simulink model "DTU_Topology_Long_Line"  (R2023b)
settings: Solver=ode4  StartTime=0.0  StopTime=stoptime  FixedStep=Ts  RelTol=1e-3
PreLoadFcn:
  | Ts=1e-4;run('Grid_Parameters_3ph.m');load('Data_3ph_Pars.mat');load('First_Busbar_Pars.mat');run('line_parameters.m')
PostLoadFcn:
  | Ts=1e-4;run('Grid_Parameters_3ph.m');load('Data_3ph_Pars.mat');load('First_Busbar_Pars.mat');run('line_parameters.m')
InitFcn:
  | Ts=1e-4;run('Grid_Parameters_3ph.m');load('Data_3ph_Pars.mat');load('First_Busbar_Pars.mat');run('line_parameters.m')
StartFcn:
  | Ts=1e-4;run('Grid_Parameters_3ph.m');load('Data_3ph_Pars.mat');load('First_Busbar_Pars.mat');run('line_parameters.m')
values from neighbouring files (symbols this model uses):
  datastart = 100    [Grid_Parameters_3ph.m]
  datastop = 700    [Grid_Parameters_3ph.m]
  fnom = 50    [Grid_Parameters_3ph.m]    (also in line_parameters.m)
  line_param = struct()    [line_parameters.m]
  t_factor = 1/acceleration    (= 1)    [Grid_Parameters_3ph.m]
  timestep_meas_data = 1    [Grid_Parameters_3ph.m]
  Vnom = 400    [Grid_Parameters_3ph.m]
undefined symbols (not defined in the file or in its folder): another_event_name, Data_3ph_Pars, First_Busbar_Pars, j, my_event_name, Newton, Raphson
libraries: spsSeriesRLCBranchLib x90, spsGroundLib x47, spsThreePhaseVIMeasurementLib x11, spsMutualInductanceLib x7, spsThreePhaseSineGeneratorLib x6, spsControlledVoltageSourceLib x3, spsControlledCurrentSourceLib x3, spsMeanLib x3, rtlab x2, spsThreePhaseSourceLib x1, spsThreePhaseSeriesRLCBranchLib x1, sps_lib x1
(part 1 of 2)
Description:
  | Model of a simple control system for use iin training.
settings Model: VariantFading=off  Creator=Alex  LastModifiedBy=obus
settings SolverCC: AlgebraicLoopSolver=TrustRegion  AutoInsertRateTranBlk=on
settings DataIOCC: LimitDataPoints=on  SaveFormat=Array  SignalLoggingSaveFormat=ModelDataLogs  SaveOutput=off  SaveTime=off  ReturnWorkspaceOutputs=off  SignalLoggingName=sigsOut
settings OptimizationCC: BlockReduction=off  BooleanDataType=off  OptimizeBlockIOStorage=off  BufferReuse=off  GlobalBufferReuse=off  ExpressionFolding=off  LocalBlockOutputs=off  InitFltsAndDblsToZero=on  LifeSpan=inf  OptimizeDataStoreBuffers=off  BusAssignmentInplaceUpdate=off
settings DebuggingCC: SaveWithParameterizedLinksMsg=none  UnderspecifiedInitializationDetection=Classic  MergeDetectMultiDrivingBlocksExec=none  SignalResolutionControl=TryResolveAllWithWarning  MultiTaskDSMMsg=warning  MultiTaskCondExecSysMsg=none  FcnCallInpInsideContextMsg=warning  UnconnectedInputMsg=warning  UnconnectedOutputMsg=warning  UnconnectedLineMsg=warning  SFUnexpectedBacktrackingDiag=warning  SFNoUnconditionalDefaultTransitionDiag=warning  SFExecutionAtInitializationDiag=none  ArithmeticOperatorsInVariantConditions=warning
settings HardwareCC: ProdBitPerPointer=32  ProdBitPerSizeT=32  ProdBitPerPtrDiffT=32  ProdLargestAtomicFloat=None  ProdIntDivRoundTo=Undefined  ProdEndianess=Unspecified  ProdWordSize=32  ProdHWDeviceType=32-bit Generic  TargetUnknown=on
settings ModelReferenceCC: EnableRefExpFcnMdlSchedulingChecks=on  PropagateSignalLabelsOutOfModel=off
settings SFSimCC: SimUseLocalCustomCode=off  CustomCodeUndefinedFunction=UseInterfaceOnly
settings RTWCC: RTWUseLocalCustomCode=off  DLArmComputeVersion=19.05
settings CodeAppCC: StateflowObjectComments=on
settings GRTTargetCC: TargetFcnLib=ansi_tfl_tmw.mat  TargetLangStandard=C89/C90 (ANSI)  CombineOutputUpdateFcns=off  GRTInterface=on
settings ConfigComp: CovMetricSettings=dw  CovSaveCumulativeToWorkspaceVar=on  CovSaveSingleToWorkspaceVar=on  CovExternalEMLEnable=off

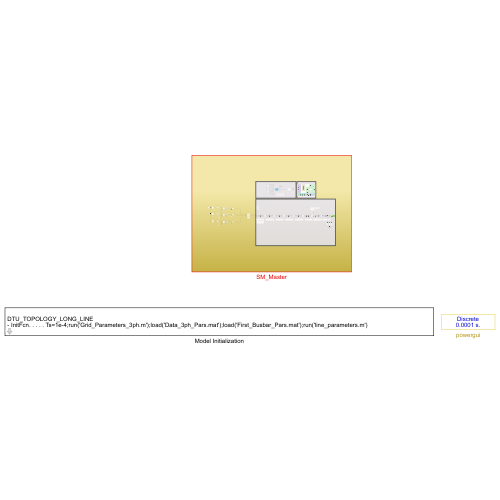
[thumbnail: Simulink's stored preview of the top-level diagram]
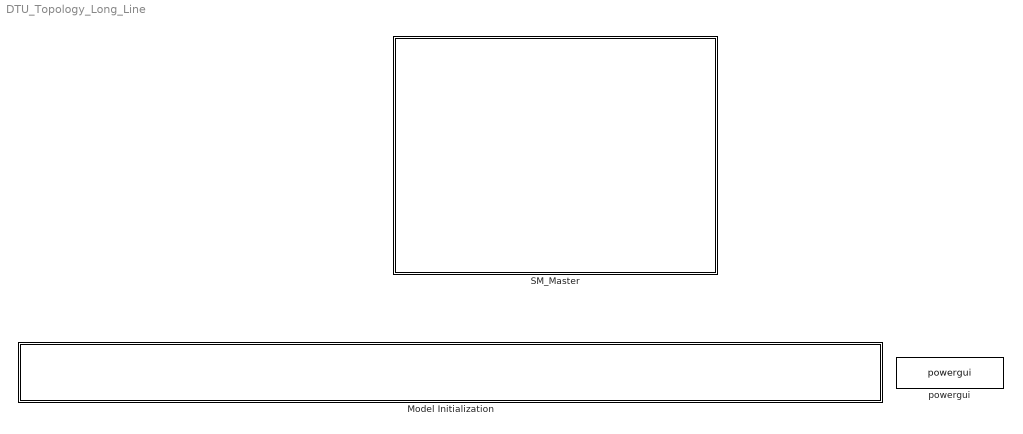
== system DTU_Topology_Long_Line ==
  Model Initialization : Subsystem  mask(Model Functions){InitFcnX=Ts=1e-4;run('Grid_Parameters_3ph.m');load('Data_3ph_Pars.mat');load('First_Busbar_Pars.mat');run('line_parameters.m'), prel=on, posl=on, inif=on, strf=on}
      mask prompts: InitFcnX "Initialisation"; prel "Preload Function"; posl "PostLoad Function"; inif "InitFcn"; strf "StartFcn"
      mask init:
      | currentBlock = gcb;
      | root = bdroot(currentBlock);
      | 
      | if ~strcmp(get_param(root,'BlockDiagramType'),'library')
      |     if prel==1
      |         set_param(root, 'PreLoadFcn', InitFcnX);
      |     else
      |         set_param(root, 'PreLoadFcn', '');
      |     end
      |     if inif==1
      |         set_param(root, 'InitFcn', InitFcnX);
      |     else
      |         set_param(root, 'InitFcn', '');
      |     end
      |     if strf==1
      |         set_param(root, 'StartFcn', InitFcnX);
      |     else
      |         set_param(root, 'StartFcn', '');
      |     end
      |     if posl==1
      |         set_param(root, 'PostLoadFcn', InitFcnX);
      |     else
      |         set_param(root, 'PostLoadFcn', '');
      |     end
      | end
      | 
      | pos = get_param(currentBlock, 'Position');
      | width = pos(3) - pos(1); height = pos(4) - pos(2);
      | txt = [ upper(root) '\n' '- InitFcn. . . . . '  get_param(root, 'InitFcn') ];
      settings: CopyFcn=set_param(gcb,'LinkStatus','none')
      mask Display: text(5, height*0.5, txt, 'horizontalAlignment', 'left', 'verticalAlignment', 'middle') ;
  SM_Master : Subsystem
  powergui : sps_lib/powergui  Priority=2  SimulationMode=Discrete  SampleTime=Ts  frequency=60  Iterations=50  frequencyindice=50  Pbase=100e6  ErrMax=1e-4  UnitsV=V  UnitsW=kW  buscounter=0  FunctionMessages=off  echomessages=off  EnableUseOfTLC=off  CurrentSourceSwitches=off  DisableSnubberDevices=off  DisableRonSwitches=off  DisableVfSwitches=off  DisplayEquations=off  AutomaticDiscreteSolvers=off  SolverType=Tustin  Interpol=off  ExternalGateDelay=off  methode=off  Ts=0  x0status=steady  SPID=off  SwTol=0  HookPort=off  NonlinearTolerance=0  nMaxIteration=15  ContinueOnMaxIteration=off  RestoreLinks=warning  ResistiveCurrentMeasurement=off  Frange=logspace(0,3,50)  Ylog=off  Xlog=off  ShowGrid=off  save=off  variable=ZData  structure=0  ZoomFFT=on  StartTime=0.0  cycles=1  DisplayStyle=1  fundamental=60  FreqAxis=off  MaxFrequency=1000  frequencyindicesteady=1  RmsSteady=2  display=off

== system DTU_Topology_Long_Line/Model Initialization ==

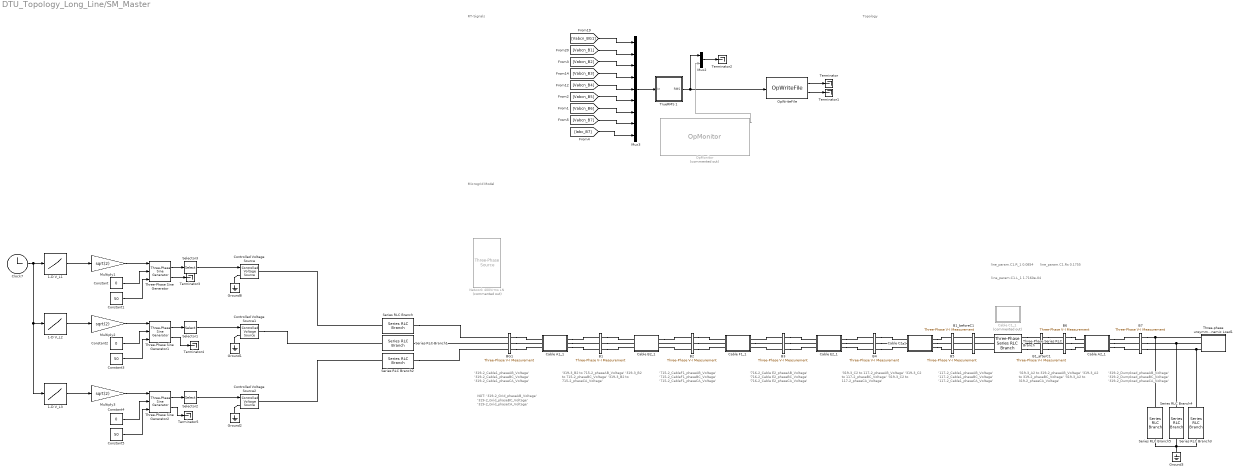
== system DTU_Topology_Long_Line/SM_Master ==
  note: line_param.C1.L_1
      | 1.7160e-04
  note: line_param.C1.Rs
      | 0.1755
  note: line_param.C1.R_1
      | 0.0854
  note: '319-2_Cable1_phaseAB_Voltage'
      | '319-2_Cable1_phaseBC_Voltage'
      | '319-2_Cable1_phaseCA_Voltage'
  note: RT-Signals
  note: Microgrid Model
  note: Topology
  note: '319-3_B2 to 715-2_phaseAB_Voltage'
      | '319-3_B2 to 715-2_phaseBC_Voltage'
      | '319-3_B2 to 715-2_phaseCA_Voltage'
  note: '715-2_CableF1_phaseAB_Voltage'
      | '715-2_CableF1_phaseBC_Voltage'
      | '715-2_CableF1_phaseCA_Voltage'
  note: '716-2_Cable E2_phaseAB_Voltage'
      | '716-2_Cable E2_phaseBC_Voltage'
      | '716-2_Cable E2_phaseCA_Voltage'
  note: '319-3_C2 to 117-2_phaseAB_Voltage'
      | '319-3_C2 to 117-2_phaseBC_Voltage'
      | '319-3_C2 to 117-2_phaseCA_Voltage'
  note: '117-2_Cable1_phaseAB_Voltage'
      | '117-2_Cable1_phaseBC_Voltage'
      | '117-2_Cable1_phaseCA_Voltage'
  note: '319-3_A2 to 319-2_phaseAB_Voltage'
      | '319-3_A2 to 319-2_phaseBC_Voltage'
      | '319-3_A2 to 319-2_phaseCA_Voltage'
  note: '319-2_Dumpload_phaseAB_Voltage'
      | '319-2_Dumpload_phaseBC_Voltage'
      | '319-2_Dumpload_phaseCA_Voltage'
  note: NOT:
      | '319-2_Grid_phaseAB_Voltage'
      | '319-2_Grid_phaseBC_Voltage'
      | '319-2_Grid_phaseCA_Voltage'
  1-D V_L1 : Lookup_n-D  NumberOfTableDimensions=1  BreakpointsForDimension1=t_factor * [0:timestep_meas_data:(First_Busbar_Pars.Time(datastop)-First_Busbar_Pars.Time(datastart))]'  Table=First_Busbar_Pars.VoltageL1(datastart:datastop)  InterpMethod=Flat  InternalRulePriority=Speed  RndMeth=Simplest
  1-D V_L2 : Lookup_n-D  NumberOfTableDimensions=1  BreakpointsForDimension1=t_factor * [0:timestep_meas_data:(First_Busbar_Pars.Time(datastop)-First_Busbar_Pars.Time(datastart))]'  Table=First_Busbar_Pars.VoltageL2(datastart:datastop)  InterpMethod=Flat  InternalRulePriority=Speed  RndMeth=Simplest
  1-D V_L3 : Lookup_n-D  NumberOfTableDimensions=1  BreakpointsForDimension1=t_factor * [0:timestep_meas_data:(First_Busbar_Pars.Time(datastop)-First_Busbar_Pars.Time(datastart))]'  Table=First_Busbar_Pars.VoltageL3(datastart:datastop)  InterpMethod=Flat  InternalRulePriority=Speed  RndMeth=Simplest
  B1 : spsThreePhaseVIMeasurementLib/Three-Phase V-I Measurement  VoltageMeasurement=phase-to-ground  SetLabelV=on  LabelV=Vabcn_B1  Vpu=off  VpuLL=off  CurrentMeasurement=no  SetLabelI=on  LabelI=Iabc_G2  Ipu=on  Pbase=900e6  Vbase=400  OutputType=Complex  PhasorSimulation=off  PSBequivalent=0
  B1_afterC1 : spsThreePhaseVIMeasurementLib/Three-Phase V-I Measurement  VoltageMeasurement=phase-to-ground  SetLabelV=on  LabelV=Vabcn_afterC1  Vpu=off  VpuLL=off  CurrentMeasurement=yes  SetLabelI=on  LabelI=Iabc_afterC1  Ipu=off  Pbase=900e6  Vbase=400  OutputType=Complex  PhasorSimulation=off  PSBequivalent=0
  B1_beforeC1 : spsThreePhaseVIMeasurementLib/Three-Phase V-I Measurement  VoltageMeasurement=phase-to-ground  SetLabelV=on  LabelV=Vabcn_beforeC1  Vpu=off  VpuLL=off  CurrentMeasurement=yes  SetLabelI=on  LabelI=Iabc_beforeC1  Ipu=off  Pbase=900e6  Vbase=400  OutputType=Complex  PhasorSimulation=off  PSBequivalent=0
  B2 : spsThreePhaseVIMeasurementLib/Three-Phase V-I Measurement  VoltageMeasurement=phase-to-ground  SetLabelV=on  LabelV=Vabcn_B2  Vpu=off  VpuLL=off  CurrentMeasurement=no  SetLabelI=on  LabelI=Iabc_G2  Ipu=on  Pbase=900e6  Vbase=400  OutputType=Complex  PhasorSimulation=off  PSBequivalent=0
  B3 : spsThreePhaseVIMeasurementLib/Three-Phase V-I Measurement  VoltageMeasurement=phase-to-ground  SetLabelV=on  LabelV=Vabcn_B3  Vpu=off  VpuLL=off  CurrentMeasurement=no  SetLabelI=on  LabelI=Iabc_G2  Ipu=on  Pbase=900e6  Vbase=400  OutputType=Complex  PhasorSimulation=off  PSBequivalent=0
  B4 : spsThreePhaseVIMeasurementLib/Three-Phase V-I Measurement  VoltageMeasurement=phase-to-ground  SetLabelV=on  LabelV=Vabcn_B4  Vpu=off  VpuLL=off  CurrentMeasurement=no  SetLabelI=on  LabelI=Iabc_G2  Ipu=on  Pbase=900e6  Vbase=400  OutputType=Complex  PhasorSimulation=off  PSBequivalent=0
  B5 : spsThreePhaseVIMeasurementLib/Three-Phase V-I Measurement  VoltageMeasurement=phase-to-ground  SetLabelV=on  LabelV=Vabcn_B5  Vpu=off  VpuLL=off  CurrentMeasurement=no  SetLabelI=on  LabelI=Iabc_G2  Ipu=on  Pbase=900e6  Vbase=400  OutputType=Complex  PhasorSimulation=off  PSBequivalent=0
  B6 : spsThreePhaseVIMeasurementLib/Three-Phase V-I Measurement  VoltageMeasurement=phase-to-ground  SetLabelV=on  LabelV=Vabcn_B6  Vpu=off  VpuLL=off  CurrentMeasurement=no  SetLabelI=on  LabelI=Iabc_G2  Ipu=on  Pbase=900e6  Vbase=400  OutputType=Complex  PhasorSimulation=off  PSBequivalent=0
  B7 : spsThreePhaseVIMeasurementLib/Three-Phase V-I Measurement  VoltageMeasurement=phase-to-ground  SetLabelV=on  LabelV=Vabcn_B7  Vpu=off  VpuLL=off  CurrentMeasurement=yes  SetLabelI=on  LabelI=Iabc_B7  Ipu=off  Pbase=900e6  Vbase=400  OutputType=Complex  PhasorSimulation=off  PSBequivalent=0
  BG1 : spsThreePhaseVIMeasurementLib/Three-Phase V-I Measurement  VoltageMeasurement=phase-to-ground  SetLabelV=on  LabelV=Vabcn_BG1  Vpu=off  VpuLL=off  CurrentMeasurement=no  SetLabelI=on  LabelI=Iabc_G2  Ipu=on  Pbase=900e6  Vbase=400  OutputType=Complex  PhasorSimulation=off  PSBequivalent=0
  Cable A1_1 : Subsystem  mask(ZHAW_Config){fNom=fnom, length=line_param.A1.length}
      mask prompts: fNom "Nominal frequency (Hz)"; length "Length (km)"
      mask Display:
      | patch([20 20 80 80], [0 20 20 0])
      | patch([0 0 20 20], [7 13 13 7])
      | patch([80 80 100 100], [7 13 13 7])
      | 
      | patch([20 20 80 80], [40 60 60 40])
      | patch([0 0 20 20], [47 53 53 47])
      | patch([80 80 100 100], [47 53 53 47])
      | 
      | patch([20 20 80 80], [80 100 100 80])
      | patch([0 0 20 20], [87 93 93 87])
      | patch([80 80 100 100], [87 93 93 87])
  Cable A2_1 : Subsystem  mask(ZHAW_Config){fNom=fnom, length=line_param.A2.length}
      mask prompts: fNom "Nominal frequency (Hz)"; length "Length (km)"
      mask Display:
      | patch([20 20 80 80], [0 20 20 0])
      | patch([0 0 20 20], [7 13 13 7])
      | patch([80 80 100 100], [7 13 13 7])
      | 
      | patch([20 20 80 80], [40 60 60 40])
      | patch([0 0 20 20], [47 53 53 47])
      | patch([80 80 100 100], [47 53 53 47])
      | 
      | patch([20 20 80 80], [80 100 100 80])
      | patch([0 0 20 20], [87 93 93 87])
      | patch([80 80 100 100], [87 93 93 87])
  Cable B2_1 : Subsystem  mask(ZHAW_Config){fNom=fnom, length=line_param.B2.length}
      mask prompts: fNom "Nominal frequency (Hz)"; length "Length (km)"
      mask Display:
      | patch([20 20 80 80], [0 20 20 0])
      | patch([0 0 20 20], [7 13 13 7])
      | patch([80 80 100 100], [7 13 13 7])
      | 
      | patch([20 20 80 80], [40 60 60 40])
      | patch([0 0 20 20], [47 53 53 47])
      | patch([80 80 100 100], [47 53 53 47])
      | 
      | patch([20 20 80 80], [80 100 100 80])
      | patch([0 0 20 20], [87 93 93 87])
      | patch([80 80 100 100], [87 93 93 87])
  Cable C1_1 : Subsystem  Commented=on  mask(ZHAW_Config){fNom=fnom, length=line_param.C1.length}
      mask prompts: fNom "Nominal frequency (Hz)"; length "Length (km)"
      mask Display:
      | patch([20 20 80 80], [0 20 20 0])
      | patch([0 0 20 20], [7 13 13 7])
      | patch([80 80 100 100], [7 13 13 7])
      | 
      | patch([20 20 80 80], [40 60 60 40])
      | patch([0 0 20 20], [47 53 53 47])
      | patch([80 80 100 100], [47 53 53 47])
      | 
      | patch([20 20 80 80], [80 100 100 80])
      | patch([0 0 20 20], [87 93 93 87])
      | patch([80 80 100 100], [87 93 93 87])
  Cable C2_1 : Subsystem  mask(ZHAW_Config){fNom=fnom, length=line_param.C2.length}
      mask prompts: fNom "Nominal frequency (Hz)"; length "Length (km)"
      mask Display:
      | patch([20 20 80 80], [0 20 20 0])
      | patch([0 0 20 20], [7 13 13 7])
      | patch([80 80 100 100], [7 13 13 7])
      | 
      | patch([20 20 80 80], [40 60 60 40])
      | patch([0 0 20 20], [47 53 53 47])
      | patch([80 80 100 100], [47 53 53 47])
      | 
      | patch([20 20 80 80], [80 100 100 80])
      | patch([0 0 20 20], [87 93 93 87])
      | patch([80 80 100 100], [87 93 93 87])
  Cable E2_1 : Subsystem  mask(ZHAW_Config){fNom=fnom, length=line_param.E2.length}
      mask prompts: fNom "Nominal frequency (Hz)"; length "Length (km)"
      mask Display:
      | patch([20 20 80 80], [0 20 20 0])
      | patch([0 0 20 20], [7 13 13 7])
      | patch([80 80 100 100], [7 13 13 7])
      | 
      | patch([20 20 80 80], [40 60 60 40])
      | patch([0 0 20 20], [47 53 53 47])
      | patch([80 80 100 100], [47 53 53 47])
      | 
      | patch([20 20 80 80], [80 100 100 80])
      | patch([0 0 20 20], [87 93 93 87])
      | patch([80 80 100 100], [87 93 93 87])
  Cable F1_1 : Subsystem  mask(ZHAW_Config){fNom=fnom, length=line_param.F1.length}
      mask prompts: fNom "Nominal frequency (Hz)"; length "Length (km)"
      mask Display:
      | patch([20 20 80 80], [0 20 20 0])
      | patch([0 0 20 20], [7 13 13 7])
      | patch([80 80 100 100], [7 13 13 7])
      | 
      | patch([20 20 80 80], [40 60 60 40])
      | patch([0 0 20 20], [47 53 53 47])
      | patch([80 80 100 100], [47 53 53 47])
      | 
      | patch([20 20 80 80], [80 100 100 80])
      | patch([0 0 20 20], [87 93 93 87])
      | patch([80 80 100 100], [87 93 93 87])
  Clock7 : Clock
  Constant : Constant  Value=0
  Constant1 : Constant  Value=50
  Constant2 : Constant  Value=0
  Constant3 : Constant  Value=50
  Constant4 : Constant  Value=0
  Constant5 : Constant  Value=50
  Controlled Voltage Source : spsControlledVoltageSourceLib/Controlled Voltage Source  Initialize=on  Source_Type=AC  Amplitude=400  Phase=0  Frequency=50  Measurements=Voltage
  Controlled Voltage Source1 : spsControlledVoltageSourceLib/Controlled Voltage Source  Initialize=on  Source_Type=AC  Amplitude=400  Phase=0  Frequency=50  Measurements=Voltage
  Controlled Voltage Source2 : spsControlledVoltageSourceLib/Controlled Voltage Source  Initialize=on  Source_Type=AC  Amplitude=400  Phase=0  Frequency=50  Measurements=Voltage
  Ground{1..3,8} (4 alike) : spsGroundLib/Ground  LConnTagsString=a
  Multiply1 : Gain  Gain=sqrt(2)
  Multiply2 : Gain  Gain=sqrt(2)
  Multiply3 : Gain  Gain=sqrt(2)
  Mux2 : Mux  Inputs=2
  Mux3 : Mux  Inputs=[3 3 3 3 3 3 3 3 3]
  "Network 400Vrms LN " : spsThreePhaseSourceLib/Three-Phase Source  Commented=on  InternalConnection=Yg  VoltagePhases=off  Voltage=400  PhaseAngle=0  Voltage_phases=[400 400 400]/sqrt(3)*1.00006  PhaseAngles_phases=[0 -120 +120]  Frequency=50  NonIdealSource=on  SpecifyImpedance=on  Resistance=400^2/10e6/10  Inductance=400^2/10e6/(2*pi*50)  ShortCircuitLevel=60e6  BaseVoltage=400  XRratio=1/0.1  BusType=swing  Pref=0  Qref=0  Prefabc=[10e3, 10e3, 10e3]  Qrefabc=[0, 0, 0]  Qmin=-Inf  Qmax=Inf
  OpMonitor : rtlab/Monitoring/OpMonitor  Commented=on  compute_time=on  real_step=on  idle_time=on  nb_overruns=on  user_time=off  user_name=my_event_name,another_event_name
      settings: SourceProductName=RT-LAB
  OpWriteFile : rtlab/DataLogging/OpWriteFile  Static_File=on  varname=DTU_03052222_seriesRL  Filename=DTU_02052222_seriesRL.mat  rtpath='./'  nrtpath='.\'  Acq_Group=26  file_size=[500e6]  write_offline=on  Sim_Mode=off  Nb_Samples=stoptime  Buffer_size=1000000
      settings: SourceProductName=RT-LAB  Decimation=10000
  Selector1 : Selector  InputPortWidth=3  IndexOptions=Index vector (dialog)  Indices=2  OutputSizes=1
  Selector2 : Selector  InputPortWidth=3  IndexOptions=Index vector (dialog)  Indices=3  OutputSizes=1
  Selector3 : Selector  InputPortWidth=3  IndexOptions=Index vector (dialog)  Indices=1  OutputSizes=1
  Series RLC Branch : spsSeriesRLCBranchLib/Series RLC Branch  LConnTagsString=__new0  RConnTagsString=__new0  BranchType=R  Resistance=1e-12  Inductance=1e-3  SetiL0=off  InitialCurrent=0  Capacitance=1e-6  Setx0=off  InitialVoltage=0  Measurements=None
  Series RLC Branch1 : spsSeriesRLCBranchLib/Series RLC Branch  LConnTagsString=__new0  RConnTagsString=__new0  BranchType=R  Resistance=1e-12  Inductance=1e-3  SetiL0=off  InitialCurrent=0  Capacitance=1e-6  Setx0=off  InitialVoltage=0  Measurements=None
  Series RLC Branch2 : spsSeriesRLCBranchLib/Series RLC Branch  LConnTagsString=__new0  RConnTagsString=__new0  BranchType=R  Resistance=1e-12  Inductance=1e-3  SetiL0=off  InitialCurrent=0  Capacitance=1e-6  Setx0=off  InitialVoltage=0  Measurements=None
  Series RLC Branch3 : spsSeriesRLCBranchLib/Series RLC Branch  LConnTagsString=__new0  RConnTagsString=__new0  BranchType=R  Resistance=1e12  Inductance=1e-3  SetiL0=off  InitialCurrent=0  Capacitance=1e-6  Setx0=off  InitialVoltage=0  Measurements=None
  Series RLC Branch4 : spsSeriesRLCBranchLib/Series RLC Branch  LConnTagsString=__new0  RConnTagsString=__new0  BranchType=R  Resistance=1e12  Inductance=1e-3  SetiL0=off  InitialCurrent=0  Capacitance=1e-6  Setx0=off  InitialVoltage=0  Measurements=None
  Series RLC Branch5 : spsSeriesRLCBranchLib/Series RLC Branch  LConnTagsString=__new0  RConnTagsString=__new0  BranchType=R  Resistance=1e12  Inductance=1e-3  SetiL0=off  InitialCurrent=0  Capacitance=1e-6  Setx0=off  InitialVoltage=0  Measurements=None
  Terminator{,1..5} (6 alike) : Terminator
  Three-Phase Series RLC Branch : spsThreePhaseSeriesRLCBranchLib/Three-Phase Series RLC Branch  LConnTagsString=A|B|C  RConnTagsString=A|B|C  BranchType=RL  Resistance=0.0854  Inductance=1.7160e-04  Capacitance=1e-6  Measurements=None
  Three-Phase Sine Generator : spsThreePhaseSineGeneratorLib/Three-Phase Sine Generator  Ts=0
      settings: LibrarySourceBlock=|
      | sps_lib/Sources/Signal Generator Sources/Three-Phase
      | Sine Generator
  Three-Phase Sine Generator1 : spsThreePhaseSineGeneratorLib/Three-Phase Sine Generator  Ts=0
      settings: LibrarySourceBlock=|
      | sps_lib/Sources/Signal Generator Sources/Three-Phase
      | Sine Generator
  Three-Phase Sine Generator2 : spsThreePhaseSineGeneratorLib/Three-Phase Sine Generator  Ts=0
      settings: LibrarySourceBlock=|
      | sps_lib/Sources/Signal Generator Sources/Three-Phase
      | Sine Generator
  Three-phase unsymmetrical Dynamic Load1 : Subsystem
  TrueRMS 1 : Subsystem  AncestorBlock=powerlib_meascontrol/Measurements/RMS/TrueRMS
  wires:
  [Vabcn_BG1] -> Mux3/1
  [Vabcn_B1] -> Mux3/2
  [Vabcn_B3] -> Mux3/4
  [Vabcn_B4] -> Mux3/5
  [Vabcn_B2] -> Mux3/3
  [Vabcn_B5] -> Mux3/6
  [Vabcn_B6] -> Mux3/7
  [Vabcn_B7] -> Mux3/8
  [Iabc_B7] -> Mux3/9
  Three-Phase Sine Generator/1 -> Selector3/1
  Three-Phase Sine Generator1/1 -> Selector1/1
  Selector1/1 -> Controlled Voltage Source1/1
  Three-Phase Sine Generator2/1 -> Selector2/1
  Constant4/1 -> Three-Phase Sine Generator2/2
  Constant3/1 -> Three-Phase Sine Generator1/3
  Multiply2/1 -> Three-Phase Sine Generator1/1
  Multiply3/1 -> Three-Phase Sine Generator2/1
  Clock7/1 -> 1-D V_L3/1, 1-D V_L2/1, 1-D V_L1/1
  1-D V_L2/1 -> Multiply2/1
  1-D V_L3/1 -> Multiply3/1
  Selector2/1 -> Controlled Voltage Source2/1
  Constant5/1 -> Three-Phase Sine Generator2/3
  Selector3/1 -> Controlled Voltage Source/1
  Constant1/1 -> Three-Phase Sine Generator/3
  Multiply1/1 -> Three-Phase Sine Generator/1
  1-D V_L1/1 -> Multiply1/1
  Constant/1 -> Three-Phase Sine Generator/2
  Constant2/1 -> Three-Phase Sine Generator1/2
  OpWriteFile/2 -> Terminator1/1
  OpWriteFile/1 -> Terminator/1
  Mux3/1 -> TrueRMS 1/1(In)
  TrueRMS 1/1(RMS) -> Mux2/1, OpWriteFile/1
  OpMonitor/1 -> Mux2/2
  Mux2/1 -> Terminator2/1
  Three-Phase Sine Generator/2 -> Terminator3/1
  Three-Phase Sine Generator1/2 -> Terminator4/1
  Three-Phase Sine Generator2/2 -> Terminator5/1
  connections:
  Ground1/LConn1 -- Controlled Voltage Source1/LConn1
  Ground2/LConn1 -- Controlled Voltage Source2/LConn1
  Ground8/LConn1 -- Controlled Voltage Source/LConn1
  Ground3/LConn1 -- Series RLC Branch3/RConn1 -- Series RLC Branch5/RConn1 -- Series RLC Branch4/RConn1
  Series RLC Branch/LConn1 -- Controlled Voltage Source/RConn1
  Controlled Voltage Source1/RConn1 -- Series RLC Branch1/LConn1
  Series RLC Branch2/LConn1 -- Controlled Voltage Source2/RConn1
  Series RLC Branch3/LConn1 -- B7/RConn3 -- Three-phase unsymmetrical Dynamic Load1/RConn3
  Series RLC Branch4/LConn1 -- B7/RConn2 -- Three-phase unsymmetrical Dynamic Load1/RConn2
  Three-phase unsymmetrical Dynamic Load1/RConn1 -- B7/RConn1 -- Series RLC Branch5/LConn1
  BG1/RConn1 -- Cable A1_1/LConn1
  BG1/RConn2 -- Cable A1_1/LConn2
  BG1/RConn3 -- Cable A1_1/LConn3
  Cable A1_1/RConn1 -- B1/LConn1
  B1/RConn1 -- Cable B2_1/LConn1
  Cable A1_1/RConn2 -- B1/LConn2
  B1/RConn2 -- Cable B2_1/LConn2
  Cable A1_1/RConn3 -- B1/LConn3
  B1/RConn3 -- Cable B2_1/LConn3
  B2/LConn2 -- Cable B2_1/RConn2
  Cable B2_1/RConn1 -- B2/LConn1
  B2/RConn1 -- Cable F1_1/LConn1
  B2/RConn2 -- Cable F1_1/LConn2
  B2/LConn3 -- Cable B2_1/RConn3
  B2/RConn3 -- Cable F1_1/LConn3
  B3/LConn1 -- Cable F1_1/RConn1
  Cable F1_1/RConn2 -- B3/LConn2
  B3/LConn3 -- Cable F1_1/RConn3
  B3/RConn1 -- Cable E2_1/LConn1
  B3/RConn2 -- Cable E2_1/LConn2
  B3/RConn3 -- Cable E2_1/LConn3
  Cable E2_1/RConn1 -- B4/LConn1
  B4/RConn1 -- Cable C2_1/LConn1
  Cable E2_1/RConn2 -- B4/LConn2
  B4/RConn2 -- Cable C2_1/LConn2
  Cable E2_1/RConn3 -- B4/LConn3
  B4/RConn3 -- Cable C2_1/LConn3
  Cable C2_1/RConn1 -- B5/LConn1
  Cable C2_1/RConn2 -- B5/LConn2
  Cable C2_1/RConn3 -- B5/LConn3
  B6/RConn1 -- Cable A2_1/LConn1
  B6/RConn2 -- Cable A2_1/LConn2
  B6/RConn3 -- Cable A2_1/LConn3
  Cable A2_1/RConn1 -- B7/LConn1
  Cable A2_1/RConn2 -- B7/LConn2
  Cable A2_1/RConn3 -- B7/LConn3
  Series RLC Branch/RConn1 -- BG1/LConn1
  BG1/LConn2 -- Series RLC Branch1/RConn1
  Series RLC Branch2/RConn1 -- BG1/LConn3
  B1_beforeC1/LConn1 -- B5/RConn1
  B1_beforeC1/LConn2 -- B5/RConn2
  B1_beforeC1/LConn3 -- B5/RConn3
  B1_afterC1/RConn1 -- B6/LConn1
  B1_afterC1/RConn2 -- B6/LConn2
  B1_afterC1/RConn3 -- B6/LConn3
  Three-Phase Series RLC Branch/LConn1 -- B1_beforeC1/RConn1
  Three-Phase Series RLC Branch/LConn2 -- B1_beforeC1/RConn2
  Three-Phase Series RLC Branch/LConn3 -- B1_beforeC1/RConn3
  Three-Phase Series RLC Branch/RConn1 -- B1_afterC1/LConn1
  Three-Phase Series RLC Branch/RConn2 -- B1_afterC1/LConn2
  Three-Phase Series RLC Branch/RConn3 -- B1_afterC1/LConn3

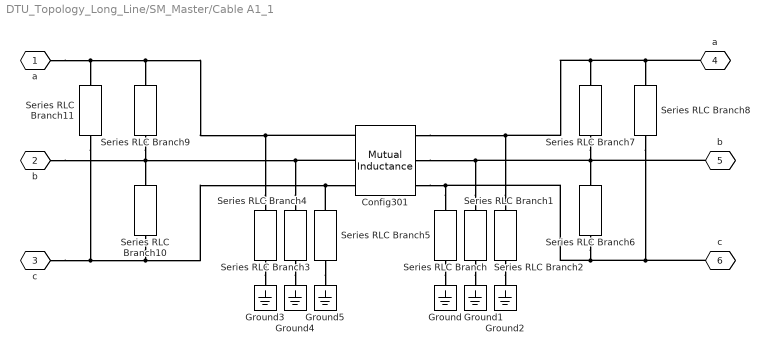
== system DTU_Topology_Long_Line/SM_Master/Cable A1_1 ==
  Config301 : spsMutualInductanceLib/Mutual Inductance  LConnTagsString=a|b|c  RConnTagsString=A|B|C  TypeOfMutual=Generalized mutual inductance  NumberOfWindings=3  SelfImpedance1=[1.1 1.1e-03]  SelfImpedance2=[ 1.1 1.1e-03]  ThreeWindings=on  SelfImpedance3=[ 1.1 1.1e-03]  MutualImpedance=[1.0 1.0e-03]  InductanceMatrix=[line_param.A1.Ls line_param.A1.Lm line_param.A1.Lm ; line_param.A1.Lm line_param.A1.Ls line_param.A1.Lm ; line_param.A1.Lm line_param.A1.Lm line_param.A1.Ls]  ResistanceMatrix=[line_param.A1.Rs line_param.A1.Rm line_param.A1.Rm ; line_param.A1.Rm line_param.A1.Rs line_param.A1.Rm ; line_param.A1.Rm line_param.A1.Rm line_param.A1.Rs]  Measurements=None
      settings: LibrarySourceBlock=sps_lib/Passives/Mutual Inductance
  Ground{,1..5} (6 alike) : spsGroundLib/Ground  LConnTagsString=a
  Series RLC Branch{,1..5} (6 alike) : spsSeriesRLCBranchLib/Series RLC Branch  LConnTagsString=__new0  RConnTagsString=__new0  BranchType=C  Resistance=1  Inductance=1e-3  SetiL0=off  InitialCurrent=0  Capacitance=line_param.A1.Cg / 2  Setx0=off  InitialVoltage=0  Measurements=None
  Series RLC Branch{6..11} (6 alike) : spsSeriesRLCBranchLib/Series RLC Branch  LConnTagsString=__new0  RConnTagsString=__new0  BranchType=C  Resistance=1  Inductance=1e-3  SetiL0=off  InitialCurrent=0  Capacitance=line_param.A1.Cp / 2  Setx0=off  InitialVoltage=0  Measurements=None
  a : PMIOPort  Tag=PMCPort  Side=Left
  b : PMIOPort  Tag=PMCPort  Port=2  Side=Left
  c : PMIOPort  Tag=PMCPort  Port=3  Side=Left
  "a " : PMIOPort  Tag=PMCPort  Port=4  Side=Right
  "b " : PMIOPort  Tag=PMCPort  Port=5  Side=Right
  "c " : PMIOPort  Tag=PMCPort  Port=6  Side=Right
  connections:
  Series RLC Branch5/RConn1 -- Ground5/LConn1
  Series RLC Branch4/RConn1 -- Ground4/LConn1
  Series RLC Branch3/RConn1 -- Ground3/LConn1
  Series RLC Branch2/RConn1 -- Ground2/LConn1
  Series RLC Branch1/RConn1 -- Ground1/LConn1
  Series RLC Branch/RConn1 -- Ground/LConn1
  Series RLC Branch/LConn1 -- Config301/RConn3 -- Series RLC Branch8/RConn1 -- "c "/RConn1 -- Series RLC Branch6/RConn1
  Series RLC Branch1/LConn1 -- Config301/RConn2 -- Series RLC Branch7/RConn1 -- Series RLC Branch6/LConn1 -- "b "/RConn1
  Series RLC Branch2/LConn1 -- Config301/RConn1 -- Series RLC Branch8/LConn1 -- "a "/RConn1 -- Series RLC Branch7/LConn1
  Series RLC Branch5/LConn1 -- Config301/LConn3 -- Series RLC Branch11/RConn1 -- c/RConn1 -- Series RLC Branch10/RConn1
  Series RLC Branch4/LConn1 -- Config301/LConn2 -- Series RLC Branch10/LConn1 -- Series RLC Branch9/RConn1 -- b/RConn1
  Series RLC Branch3/LConn1 -- Config301/LConn1 -- Series RLC Branch11/LConn1 -- a/RConn1 -- Series RLC Branch9/LConn1

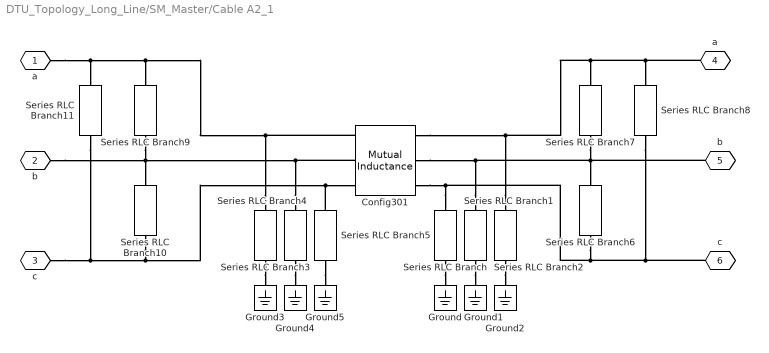
== system DTU_Topology_Long_Line/SM_Master/Cable A2_1 ==
  Config301 : spsMutualInductanceLib/Mutual Inductance  LConnTagsString=a|b|c  RConnTagsString=A|B|C  TypeOfMutual=Generalized mutual inductance  NumberOfWindings=3  SelfImpedance1=[1.1 1.1e-03]  SelfImpedance2=[ 1.1 1.1e-03]  ThreeWindings=on  SelfImpedance3=[ 1.1 1.1e-03]  MutualImpedance=[1.0 1.0e-03]  InductanceMatrix=[line_param.A2.Ls line_param.A2.Lm line_param.A2.Lm ; line_param.A2.Lm line_param.A2.Ls line_param.A2.Lm ; line_param.A2.Lm line_param.A2.Lm line_param.A2.Ls]  ResistanceMatrix=[line_param.A2.Rs line_param.A2.Rm line_param.A2.Rm ; line_param.A2.Rm line_param.A2.Rs line_param.A2.Rm ; line_param.A2.Rm line_param.A2.Rm line_param.A2.Rs]  Measurements=None
      settings: LibrarySourceBlock=sps_lib/Passives/Mutual Inductance
  Ground{,1..5} (6 alike) : spsGroundLib/Ground  LConnTagsString=a
  Series RLC Branch{,1..5} (6 alike) : spsSeriesRLCBranchLib/Series RLC Branch  LConnTagsString=__new0  RConnTagsString=__new0  BranchType=C  Resistance=1  Inductance=1e-3  SetiL0=off  InitialCurrent=0  Capacitance=line_param.A2.Cg / 2  Setx0=off  InitialVoltage=0  Measurements=None
  Series RLC Branch{6..11} (6 alike) : spsSeriesRLCBranchLib/Series RLC Branch  LConnTagsString=__new0  RConnTagsString=__new0  BranchType=C  Resistance=1  Inductance=1e-3  SetiL0=off  InitialCurrent=0  Capacitance=line_param.A2.Cp / 2  Setx0=off  InitialVoltage=0  Measurements=None
  a : PMIOPort  Tag=PMCPort  Side=Left
  b : PMIOPort  Tag=PMCPort  Port=2  Side=Left
  c : PMIOPort  Tag=PMCPort  Port=3  Side=Left
  "a " : PMIOPort  Tag=PMCPort  Port=4  Side=Right
  "b " : PMIOPort  Tag=PMCPort  Port=5  Side=Right
  "c " : PMIOPort  Tag=PMCPort  Port=6  Side=Right
  connections:
  Series RLC Branch5/RConn1 -- Ground5/LConn1
  Series RLC Branch4/RConn1 -- Ground4/LConn1
  Series RLC Branch3/RConn1 -- Ground3/LConn1
  Series RLC Branch2/RConn1 -- Ground2/LConn1
  Series RLC Branch1/RConn1 -- Ground1/LConn1
  Series RLC Branch/RConn1 -- Ground/LConn1
  Series RLC Branch/LConn1 -- Config301/RConn3 -- Series RLC Branch8/RConn1 -- "c "/RConn1 -- Series RLC Branch6/RConn1
  Series RLC Branch1/LConn1 -- Config301/RConn2 -- Series RLC Branch7/RConn1 -- Series RLC Branch6/LConn1 -- "b "/RConn1
  Series RLC Branch2/LConn1 -- Config301/RConn1 -- Series RLC Branch8/LConn1 -- "a "/RConn1 -- Series RLC Branch7/LConn1
  Series RLC Branch5/LConn1 -- Config301/LConn3 -- Series RLC Branch11/RConn1 -- c/RConn1 -- Series RLC Branch10/RConn1
  Series RLC Branch4/LConn1 -- Config301/LConn2 -- Series RLC Branch10/LConn1 -- Series RLC Branch9/RConn1 -- b/RConn1
  Series RLC Branch3/LConn1 -- Config301/LConn1 -- Series RLC Branch11/LConn1 -- a/RConn1 -- Series RLC Branch9/LConn1

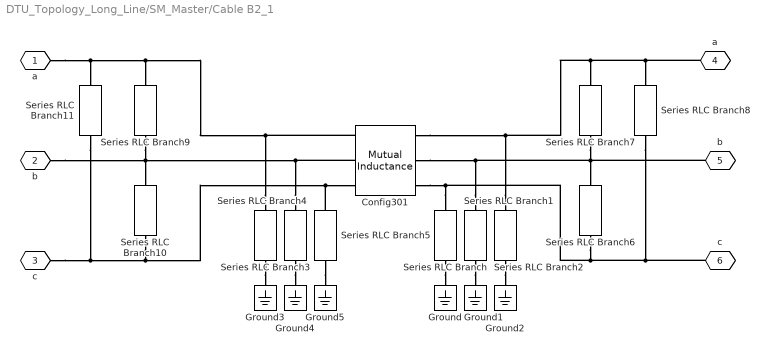
== system DTU_Topology_Long_Line/SM_Master/Cable B2_1 ==
  Config301 : spsMutualInductanceLib/Mutual Inductance  LConnTagsString=a|b|c  RConnTagsString=A|B|C  TypeOfMutual=Generalized mutual inductance  NumberOfWindings=3  SelfImpedance1=[1.1 1.1e-03]  SelfImpedance2=[ 1.1 1.1e-03]  ThreeWindings=on  SelfImpedance3=[ 1.1 1.1e-03]  MutualImpedance=[1.0 1.0e-03]  InductanceMatrix=[line_param.B2.Ls line_param.B2.Lm line_param.B2.Lm ; line_param.B2.Lm line_param.B2.Ls line_param.B2.Lm ; line_param.B2.Lm line_param.B2.Lm line_param.B2.Ls]  ResistanceMatrix=[line_param.B2.Rs line_param.B2.Rm line_param.B2.Rm ; line_param.B2.Rm line_param.B2.Rs line_param.B2.Rm ; line_param.B2.Rm line_param.B2.Rm line_param.B2.Rs]  Measurements=None
      settings: LibrarySourceBlock=sps_lib/Passives/Mutual Inductance
  Ground{,1..5} (6 alike) : spsGroundLib/Ground  LConnTagsString=a
  Series RLC Branch{,1..5} (6 alike) : spsSeriesRLCBranchLib/Series RLC Branch  LConnTagsString=__new0  RConnTagsString=__new0  BranchType=C  Resistance=1  Inductance=1e-3  SetiL0=off  InitialCurrent=0  Capacitance=line_param.B2.Cg / 2  Setx0=off  InitialVoltage=0  Measurements=None
  Series RLC Branch{6..11} (6 alike) : spsSeriesRLCBranchLib/Series RLC Branch  LConnTagsString=__new0  RConnTagsString=__new0  BranchType=C  Resistance=1  Inductance=1e-3  SetiL0=off  InitialCurrent=0  Capacitance=line_param.B2.Cp / 2  Setx0=off  InitialVoltage=0  Measurements=None
  a : PMIOPort  Tag=PMCPort  Side=Left
  b : PMIOPort  Tag=PMCPort  Port=2  Side=Left
  c : PMIOPort  Tag=PMCPort  Port=3  Side=Left
  "a " : PMIOPort  Tag=PMCPort  Port=4  Side=Right
  "b " : PMIOPort  Tag=PMCPort  Port=5  Side=Right
  "c " : PMIOPort  Tag=PMCPort  Port=6  Side=Right
  connections:
  Series RLC Branch5/RConn1 -- Ground5/LConn1
  Series RLC Branch4/RConn1 -- Ground4/LConn1
  Series RLC Branch3/RConn1 -- Ground3/LConn1
  Series RLC Branch2/RConn1 -- Ground2/LConn1
  Series RLC Branch1/RConn1 -- Ground1/LConn1
  Series RLC Branch/RConn1 -- Ground/LConn1
  Series RLC Branch/LConn1 -- Config301/RConn3 -- Series RLC Branch8/RConn1 -- "c "/RConn1 -- Series RLC Branch6/RConn1
  Series RLC Branch1/LConn1 -- Config301/RConn2 -- Series RLC Branch7/RConn1 -- Series RLC Branch6/LConn1 -- "b "/RConn1
  Series RLC Branch2/LConn1 -- Config301/RConn1 -- Series RLC Branch8/LConn1 -- "a "/RConn1 -- Series RLC Branch7/LConn1
  Series RLC Branch5/LConn1 -- Config301/LConn3 -- Series RLC Branch11/RConn1 -- c/RConn1 -- Series RLC Branch10/RConn1
  Series RLC Branch4/LConn1 -- Config301/LConn2 -- Series RLC Branch10/LConn1 -- Series RLC Branch9/RConn1 -- b/RConn1
  Series RLC Branch3/LConn1 -- Config301/LConn1 -- Series RLC Branch11/LConn1 -- a/RConn1 -- Series RLC Branch9/LConn1

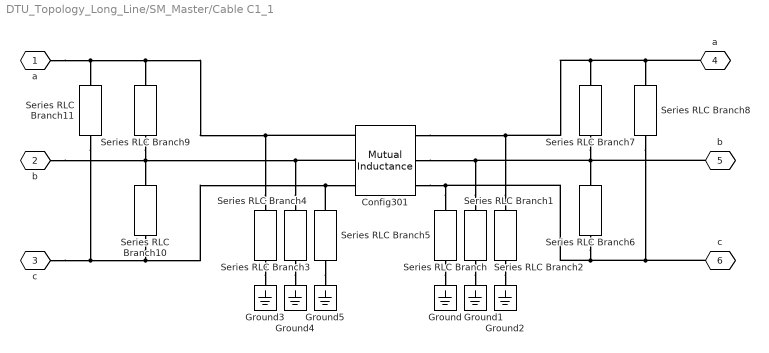
== system DTU_Topology_Long_Line/SM_Master/Cable C1_1 ==
  Config301 : spsMutualInductanceLib/Mutual Inductance  LConnTagsString=a|b|c  RConnTagsString=A|B|C  TypeOfMutual=Generalized mutual inductance  NumberOfWindings=3  SelfImpedance1=[1.1 1.1e-03]  SelfImpedance2=[ 1.1 1.1e-03]  ThreeWindings=on  SelfImpedance3=[ 1.1 1.1e-03]  MutualImpedance=[1.0 1.0e-03]  InductanceMatrix=[line_param.C1.Ls line_param.C1.Lm line_param.C1.Lm ; line_param.C1.Lm line_param.C1.Ls line_param.C1.Lm ; line_param.C1.Lm line_param.C1.Lm line_param.C1.Ls]  ResistanceMatrix=[line_param.C1.Rs line_param.C1.Rm line_param.C1.Rm ; line_param.C1.Rm line_param.C1.Rs line_param.C1.Rm ; line_param.C1.Rm line_param.C1.Rm line_param.C1.Rs]  Measurements=None
      settings: LibrarySourceBlock=sps_lib/Passives/Mutual Inductance
  Ground{,1..5} (6 alike) : spsGroundLib/Ground  LConnTagsString=a
  Series RLC Branch{,1..5} (6 alike) : spsSeriesRLCBranchLib/Series RLC Branch  LConnTagsString=__new0  RConnTagsString=__new0  BranchType=C  Resistance=1  Inductance=1e-3  SetiL0=off  InitialCurrent=0  Capacitance=line_param.C1.Cg / 2  Setx0=off  InitialVoltage=0  Measurements=None
  Series RLC Branch{6..11} (6 alike) : spsSeriesRLCBranchLib/Series RLC Branch  LConnTagsString=__new0  RConnTagsString=__new0  BranchType=C  Resistance=1  Inductance=1e-3  SetiL0=off  InitialCurrent=0  Capacitance=line_param.C1.Cp / 2  Setx0=off  InitialVoltage=0  Measurements=None
  a : PMIOPort  Tag=PMCPort  Side=Left
  b : PMIOPort  Tag=PMCPort  Port=2  Side=Left
  c : PMIOPort  Tag=PMCPort  Port=3  Side=Left
  "a " : PMIOPort  Tag=PMCPort  Port=4  Side=Right
  "b " : PMIOPort  Tag=PMCPort  Port=5  Side=Right
  "c " : PMIOPort  Tag=PMCPort  Port=6  Side=Right
  connections:
  Series RLC Branch5/RConn1 -- Ground5/LConn1
  Series RLC Branch4/RConn1 -- Ground4/LConn1
  Series RLC Branch3/RConn1 -- Ground3/LConn1
  Series RLC Branch2/RConn1 -- Ground2/LConn1
  Series RLC Branch1/RConn1 -- Ground1/LConn1
  Series RLC Branch/RConn1 -- Ground/LConn1
  Series RLC Branch/LConn1 -- Config301/RConn3 -- Series RLC Branch8/RConn1 -- "c "/RConn1 -- Series RLC Branch6/RConn1
  Series RLC Branch1/LConn1 -- Config301/RConn2 -- Series RLC Branch7/RConn1 -- Series RLC Branch6/LConn1 -- "b "/RConn1
  Series RLC Branch2/LConn1 -- Config301/RConn1 -- Series RLC Branch8/LConn1 -- "a "/RConn1 -- Series RLC Branch7/LConn1
  Series RLC Branch5/LConn1 -- Config301/LConn3 -- Series RLC Branch11/RConn1 -- c/RConn1 -- Series RLC Branch10/RConn1
  Series RLC Branch4/LConn1 -- Config301/LConn2 -- Series RLC Branch10/LConn1 -- Series RLC Branch9/RConn1 -- b/RConn1
  Series RLC Branch3/LConn1 -- Config301/LConn1 -- Series RLC Branch11/LConn1 -- a/RConn1 -- Series RLC Branch9/LConn1

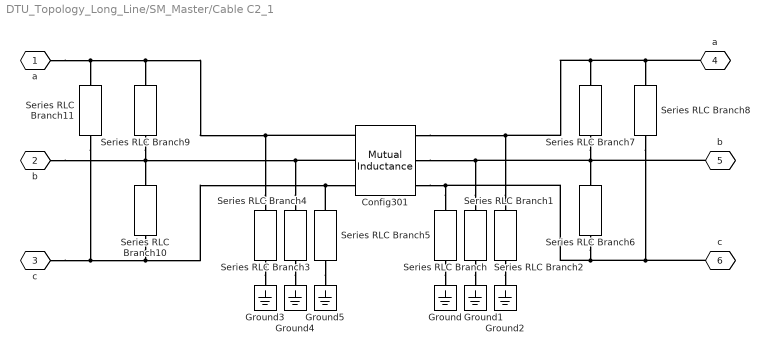
== system DTU_Topology_Long_Line/SM_Master/Cable C2_1 ==
  Config301 : spsMutualInductanceLib/Mutual Inductance  LConnTagsString=a|b|c  RConnTagsString=A|B|C  TypeOfMutual=Generalized mutual inductance  NumberOfWindings=3  SelfImpedance1=[1.1 1.1e-03]  SelfImpedance2=[ 1.1 1.1e-03]  ThreeWindings=on  SelfImpedance3=[ 1.1 1.1e-03]  MutualImpedance=[1.0 1.0e-03]  InductanceMatrix=[line_param.C2.Ls line_param.C2.Lm line_param.C2.Lm ; line_param.C2.Lm line_param.C2.Ls line_param.C2.Lm ; line_param.C2.Lm line_param.C2.Lm line_param.C2.Ls]  ResistanceMatrix=[line_param.C2.Rs line_param.C2.Rm line_param.C2.Rm ; line_param.C2.Rm line_param.C2.Rs line_param.C2.Rm ; line_param.C2.Rm line_param.C2.Rm line_param.C2.Rs]  Measurements=None
      settings: LibrarySourceBlock=sps_lib/Passives/Mutual Inductance
  Ground{,1..5} (6 alike) : spsGroundLib/Ground  LConnTagsString=a
  Series RLC Branch{,1..5} (6 alike) : spsSeriesRLCBranchLib/Series RLC Branch  LConnTagsString=__new0  RConnTagsString=__new0  BranchType=C  Resistance=1  Inductance=1e-3  SetiL0=off  InitialCurrent=0  Capacitance=line_param.C2.Cg / 2  Setx0=off  InitialVoltage=0  Measurements=None
  Series RLC Branch{6..11} (6 alike) : spsSeriesRLCBranchLib/Series RLC Branch  LConnTagsString=__new0  RConnTagsString=__new0  BranchType=C  Resistance=1  Inductance=1e-3  SetiL0=off  InitialCurrent=0  Capacitance=line_param.C2.Cp / 2  Setx0=off  InitialVoltage=0  Measurements=None
  a : PMIOPort  Tag=PMCPort  Side=Left
  b : PMIOPort  Tag=PMCPort  Port=2  Side=Left
  c : PMIOPort  Tag=PMCPort  Port=3  Side=Left
  "a " : PMIOPort  Tag=PMCPort  Port=4  Side=Right
  "b " : PMIOPort  Tag=PMCPort  Port=5  Side=Right
  "c " : PMIOPort  Tag=PMCPort  Port=6  Side=Right
  connections:
  Series RLC Branch5/RConn1 -- Ground5/LConn1
  Series RLC Branch4/RConn1 -- Ground4/LConn1
  Series RLC Branch3/RConn1 -- Ground3/LConn1
  Series RLC Branch2/RConn1 -- Ground2/LConn1
  Series RLC Branch1/RConn1 -- Ground1/LConn1
  Series RLC Branch/RConn1 -- Ground/LConn1
  Series RLC Branch/LConn1 -- Config301/RConn3 -- Series RLC Branch8/RConn1 -- "c "/RConn1 -- Series RLC Branch6/RConn1
  Series RLC Branch1/LConn1 -- Config301/RConn2 -- Series RLC Branch7/RConn1 -- Series RLC Branch6/LConn1 -- "b "/RConn1
  Series RLC Branch2/LConn1 -- Config301/RConn1 -- Series RLC Branch8/LConn1 -- "a "/RConn1 -- Series RLC Branch7/LConn1
  Series RLC Branch5/LConn1 -- Config301/LConn3 -- Series RLC Branch11/RConn1 -- c/RConn1 -- Series RLC Branch10/RConn1
  Series RLC Branch4/LConn1 -- Config301/LConn2 -- Series RLC Branch10/LConn1 -- Series RLC Branch9/RConn1 -- b/RConn1
  Series RLC Branch3/LConn1 -- Config301/LConn1 -- Series RLC Branch11/LConn1 -- a/RConn1 -- Series RLC Branch9/LConn1

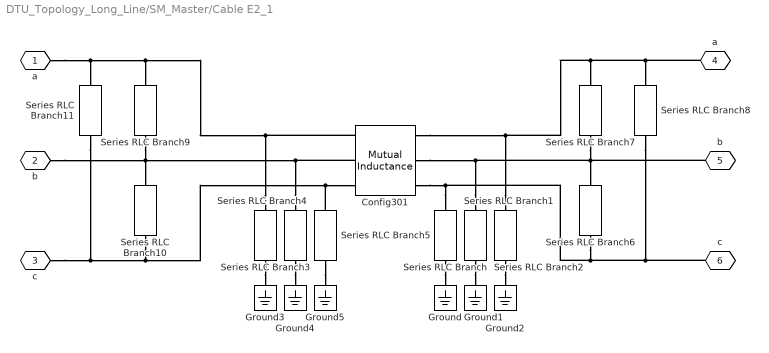
== system DTU_Topology_Long_Line/SM_Master/Cable E2_1 ==
  Config301 : spsMutualInductanceLib/Mutual Inductance  LConnTagsString=a|b|c  RConnTagsString=A|B|C  TypeOfMutual=Generalized mutual inductance  NumberOfWindings=3  SelfImpedance1=[1.1 1.1e-03]  SelfImpedance2=[ 1.1 1.1e-03]  ThreeWindings=on  SelfImpedance3=[ 1.1 1.1e-03]  MutualImpedance=[1.0 1.0e-03]  InductanceMatrix=[line_param.E2.Ls line_param.E2.Lm line_param.E2.Lm ; line_param.E2.Lm line_param.E2.Ls line_param.E2.Lm ; line_param.E2.Lm line_param.E2.Lm line_param.E2.Ls]  ResistanceMatrix=[line_param.E2.Rs line_param.E2.Rm line_param.E2.Rm ; line_param.E2.Rm line_param.E2.Rs line_param.E2.Rm ; line_param.E2.Rm line_param.E2.Rm line_param.E2.Rs]  Measurements=None
      settings: LibrarySourceBlock=sps_lib/Passives/Mutual Inductance
  Ground{,1..5} (6 alike) : spsGroundLib/Ground  LConnTagsString=a
  Series RLC Branch{,1..5} (6 alike) : spsSeriesRLCBranchLib/Series RLC Branch  LConnTagsString=__new0  RConnTagsString=__new0  BranchType=C  Resistance=1  Inductance=1e-3  SetiL0=off  InitialCurrent=0  Capacitance=line_param.E2.Cg / 2  Setx0=off  InitialVoltage=0  Measurements=None
  Series RLC Branch{6..11} (6 alike) : spsSeriesRLCBranchLib/Series RLC Branch  LConnTagsString=__new0  RConnTagsString=__new0  BranchType=C  Resistance=1  Inductance=1e-3  SetiL0=off  InitialCurrent=0  Capacitance=line_param.E2.Cp / 2  Setx0=off  InitialVoltage=0  Measurements=None
  a : PMIOPort  Tag=PMCPort  Side=Left
  b : PMIOPort  Tag=PMCPort  Port=2  Side=Left
  c : PMIOPort  Tag=PMCPort  Port=3  Side=Left
  "a " : PMIOPort  Tag=PMCPort  Port=4  Side=Right
  "b " : PMIOPort  Tag=PMCPort  Port=5  Side=Right
  "c " : PMIOPort  Tag=PMCPort  Port=6  Side=Right
  connections:
  Series RLC Branch5/RConn1 -- Ground5/LConn1
  Series RLC Branch4/RConn1 -- Ground4/LConn1
  Series RLC Branch3/RConn1 -- Ground3/LConn1
  Series RLC Branch2/RConn1 -- Ground2/LConn1
  Series RLC Branch1/RConn1 -- Ground1/LConn1
  Series RLC Branch/RConn1 -- Ground/LConn1
  Series RLC Branch/LConn1 -- Config301/RConn3 -- Series RLC Branch8/RConn1 -- "c "/RConn1 -- Series RLC Branch6/RConn1
  Series RLC Branch1/LConn1 -- Config301/RConn2 -- Series RLC Branch7/RConn1 -- Series RLC Branch6/LConn1 -- "b "/RConn1
  Series RLC Branch2/LConn1 -- Config301/RConn1 -- Series RLC Branch8/LConn1 -- "a "/RConn1 -- Series RLC Branch7/LConn1
  Series RLC Branch5/LConn1 -- Config301/LConn3 -- Series RLC Branch11/RConn1 -- c/RConn1 -- Series RLC Branch10/RConn1
  Series RLC Branch4/LConn1 -- Config301/LConn2 -- Series RLC Branch10/LConn1 -- Series RLC Branch9/RConn1 -- b/RConn1
  Series RLC Branch3/LConn1 -- Config301/LConn1 -- Series RLC Branch11/LConn1 -- a/RConn1 -- Series RLC Branch9/LConn1

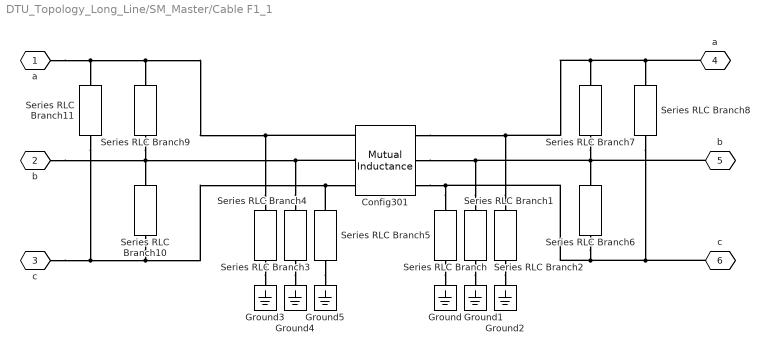
== system DTU_Topology_Long_Line/SM_Master/Cable F1_1 ==
  Config301 : spsMutualInductanceLib/Mutual Inductance  LConnTagsString=a|b|c  RConnTagsString=A|B|C  TypeOfMutual=Generalized mutual inductance  NumberOfWindings=3  SelfImpedance1=[1.1 1.1e-03]  SelfImpedance2=[ 1.1 1.1e-03]  ThreeWindings=on  SelfImpedance3=[ 1.1 1.1e-03]  MutualImpedance=[1.0 1.0e-03]  InductanceMatrix=[line_param.F1.Ls line_param.F1.Lm line_param.F1.Lm ; line_param.F1.Lm line_param.F1.Ls line_param.F1.Lm ; line_param.F1.Lm line_param.F1.Lm line_param.F1.Ls]  ResistanceMatrix=[line_param.F1.Rs line_param.F1.Rm line_param.F1.Rm ; line_param.F1.Rm line_param.F1.Rs line_param.F1.Rm ; line_param.F1.Rm line_param.F1.Rm line_param.F1.Rs]  Measurements=None
      settings: LibrarySourceBlock=sps_lib/Passives/Mutual Inductance
  Ground{,1..5} (6 alike) : spsGroundLib/Ground  LConnTagsString=a
  Series RLC Branch{,1..5} (6 alike) : spsSeriesRLCBranchLib/Series RLC Branch  LConnTagsString=__new0  RConnTagsString=__new0  BranchType=C  Resistance=1  Inductance=1e-3  SetiL0=off  InitialCurrent=0  Capacitance=line_param.F1.Cg / 2  Setx0=off  InitialVoltage=0  Measurements=None
  Series RLC Branch{6..11} (6 alike) : spsSeriesRLCBranchLib/Series RLC Branch  LConnTagsString=__new0  RConnTagsString=__new0  BranchType=C  Resistance=1  Inductance=1e-3  SetiL0=off  InitialCurrent=0  Capacitance=line_param.F1.Cp / 2  Setx0=off  InitialVoltage=0  Measurements=None
  a : PMIOPort  Tag=PMCPort  Side=Left
  b : PMIOPort  Tag=PMCPort  Port=2  Side=Left
  c : PMIOPort  Tag=PMCPort  Port=3  Side=Left
  "a " : PMIOPort  Tag=PMCPort  Port=4  Side=Right
  "b " : PMIOPort  Tag=PMCPort  Port=5  Side=Right
  "c " : PMIOPort  Tag=PMCPort  Port=6  Side=Right
  connections:
  Series RLC Branch5/RConn1 -- Ground5/LConn1
  Series RLC Branch4/RConn1 -- Ground4/LConn1
  Series RLC Branch3/RConn1 -- Ground3/LConn1
  Series RLC Branch2/RConn1 -- Ground2/LConn1
  Series RLC Branch1/RConn1 -- Ground1/LConn1
  Series RLC Branch/RConn1 -- Ground/LConn1
  Series RLC Branch/LConn1 -- Config301/RConn3 -- Series RLC Branch8/RConn1 -- "c "/RConn1 -- Series RLC Branch6/RConn1
  Series RLC Branch1/LConn1 -- Config301/RConn2 -- Series RLC Branch7/RConn1 -- Series RLC Branch6/LConn1 -- "b "/RConn1
  Series RLC Branch2/LConn1 -- Config301/RConn1 -- Series RLC Branch8/LConn1 -- "a "/RConn1 -- Series RLC Branch7/LConn1
  Series RLC Branch5/LConn1 -- Config301/LConn3 -- Series RLC Branch11/RConn1 -- c/RConn1 -- Series RLC Branch10/RConn1
  Series RLC Branch4/LConn1 -- Config301/LConn2 -- Series RLC Branch10/LConn1 -- Series RLC Branch9/RConn1 -- b/RConn1
  Series RLC Branch3/LConn1 -- Config301/LConn1 -- Series RLC Branch11/LConn1 -- a/RConn1 -- Series RLC Branch9/LConn1
